simulink model "easy_sliding_mode_1"  (R2019b)
settings: Solver=VariableStepAuto  StartTime=0.0  StopTime=10.0  RelTol=1e-3
settings Model: Creator=Alien  LastModifiedBy=Alien
settings SolverCC: ZeroCrossAlgorithm=Adaptive
settings DebuggingCC: IgnoredZcDiagnostic=none

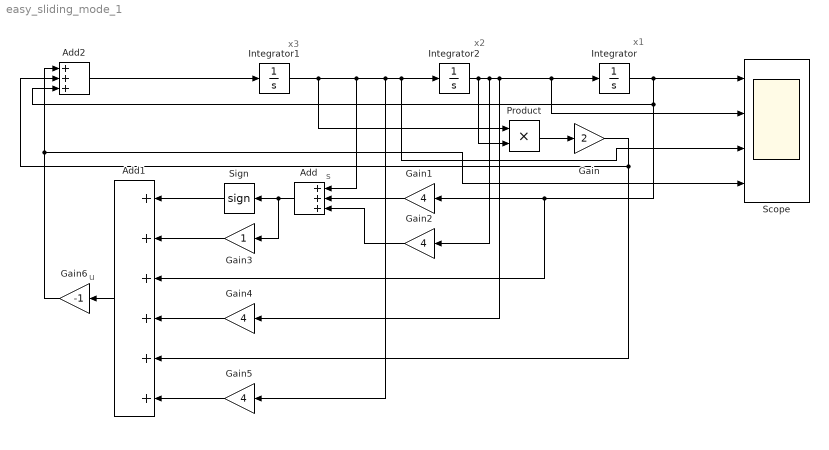
== system easy_sliding_mode_1 ==
  note: u
  note: s
  note: x3
  note: x2
  note: x1
  Add : Sum  Inputs=+++
  Add1 : Sum  Inputs=++++++
  Add2 : Sum  Inputs=+++
  Gain : Gain  Gain=2
  Gain{1..2,4..5} (4 alike) : Gain  Gain=4
  Gain3 : Gain
  Gain6 : Gain  Gain=-1
  Integrator : Integrator  InitialCondition=5
  Integrator1 : Integrator  InitialCondition=2
  Integrator2 : Integrator  InitialCondition=71
  Product : Product
  Scope : Scope  NumInputPorts=4
  Sign : Signum
  wires:
  Integrator2/1 -> Product/2, Gain4/1, Scope/2, Integrator/1, Gain2/1
  Integrator1/1 -> Product/1, Add/1, Gain5/1, Scope/3, Integrator2/1
  Product/1 -> Gain/1
  Integrator/1 -> Scope/1, Add2/3, Add1/3, Gain1/1
  Gain1/1 -> Add/2
  Gain2/1 -> Add/3
  Add/1 -> Gain3/1, Sign/1
  Sign/1 -> Add1/1
  Gain3/1 -> Add1/2
  Gain4/1 -> Add1/4
  Gain/1 -> Add2/2, Add1/5
  Gain5/1 -> Add1/6
  Add1/1 -> Gain6/1
  Add2/1 -> Integrator1/1
  Gain6/1 -> Scope/4, Add2/1
